simulink model "multi_casadi_robot"  (R2019b)
settings: Solver=FixedStepAuto  StartTime=0.0  StopTime=100  RelTol=1e-3
settings Model: Creator=sanim  LastModifiedBy=Dell
settings DataIOCC: ReturnWorkspaceOutputs=off
settings DebuggingCC: ArithmeticOperatorsInVariantConditions=warning
settings SFSimCC: CustomCodeUndefinedFunction=UseInterfaceOnly

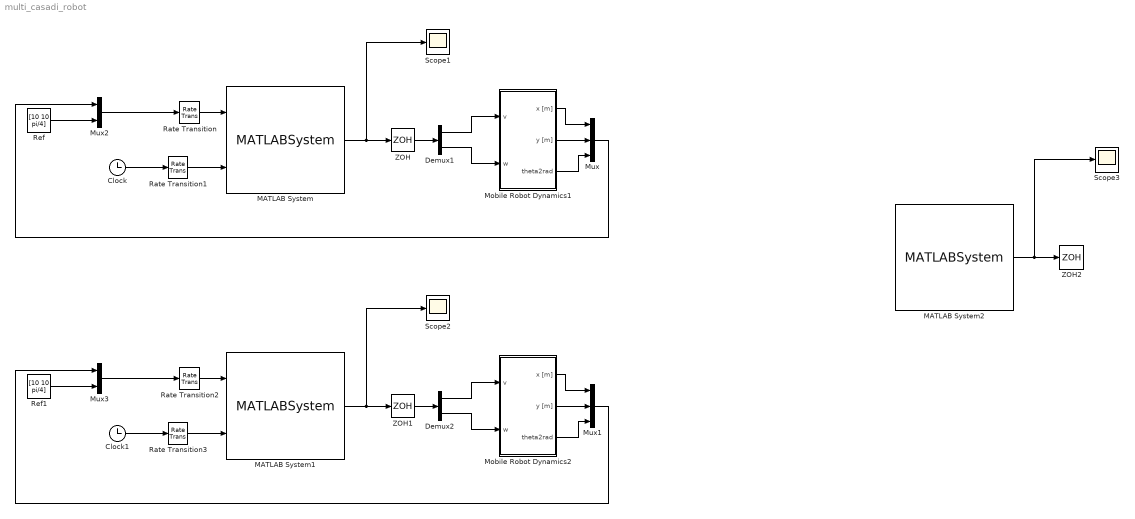
== system multi_casadi_robot ==
  Clock : Clock
  Clock1 : Clock
  Demux1 : Demux  Outputs=2
  Demux2 : Demux  Outputs=2
  MATLAB System : MATLABSystem  System=controller  SimulateUsing=Interpreted execution
      mask Type: controller
      mask Display:
      | disp('controller');
      | port_label('input',1,'x');
      | port_label('input',2,'t');
      | port_label('output',1,'u');
  MATLAB System1 : MATLABSystem  System=controller  SimulateUsing=Interpreted execution
      mask Type: controller
      mask Display:
      | disp('controller');
      | port_label('input',1,'x');
      | port_label('input',2,'t');
      | port_label('output',1,'u');
  MATLAB System2 : MATLABSystem  System=controller  SimulateUsing=Interpreted execution
      mask Type: controller
      mask Display:
      | disp('controller');
      | port_label('input',1,'x');
      | port_label('input',2,'t');
      | port_label('output',1,'u');
  Mobile Robot Dynamics1 : Subsystem
  Mobile Robot Dynamics2 : Subsystem
  Mux : Mux  Inputs=3
  Mux1 : Mux  Inputs=3
  Mux2 : Mux  Inputs=2
  Mux3 : Mux  Inputs=2
  Rate Transition{,1..3} (4 alike) : RateTransition  OutPortSampleTime=0.5
  Ref : Constant  Value=[10 10 pi/4]
  Ref1 : Constant  Value=[10 10 pi/4]
  Scope1 : Scope
  Scope2 : Scope
  Scope3 : Scope
  ZOH : ZeroOrderHold  SampleTime=0.5
  ZOH1 : ZeroOrderHold  SampleTime=0.5
  ZOH2 : ZeroOrderHold  SampleTime=0.5
  wires:
  Mobile Robot Dynamics1/2(y [m]) -> Mux/2
  ZOH/1 -> Demux1/1
  Mux/1 -> Mux2/1
  Ref/1 -> Mux2/2
  Rate Transition/1 -> MATLAB System/1
  MATLAB System/1 -> Scope1/1, ZOH/1
  Demux1/1 -> Mobile Robot Dynamics1/1(v)
  Mobile Robot Dynamics1/3(theta2rad) -> Mux/3
  Mobile Robot Dynamics1/1(x [m]) -> Mux/1
  Rate Transition1/1 -> MATLAB System/2
  Demux1/2 -> Mobile Robot Dynamics1/2(w)
  Clock/1 -> Rate Transition1/1
  Mux2/1 -> Rate Transition/1
  ZOH1/1 -> Demux2/1
  Clock1/1 -> Rate Transition3/1
  Ref1/1 -> Mux3/2
  MATLAB System1/1 -> Scope2/1, ZOH1/1
  Mobile Robot Dynamics2/1(x [m]) -> Mux1/1
  Demux2/1 -> Mobile Robot Dynamics2/1(v)
  Mobile Robot Dynamics2/3(theta2rad) -> Mux1/3
  Mux3/1 -> Rate Transition2/1
  Mux1/1 -> Mux3/1
  Rate Transition2/1 -> MATLAB System1/1
  Rate Transition3/1 -> MATLAB System1/2
  Mobile Robot Dynamics2/2(y [m]) -> Mux1/2
  Demux2/2 -> Mobile Robot Dynamics2/2(w)
  MATLAB System2/1 -> Scope3/1, ZOH2/1

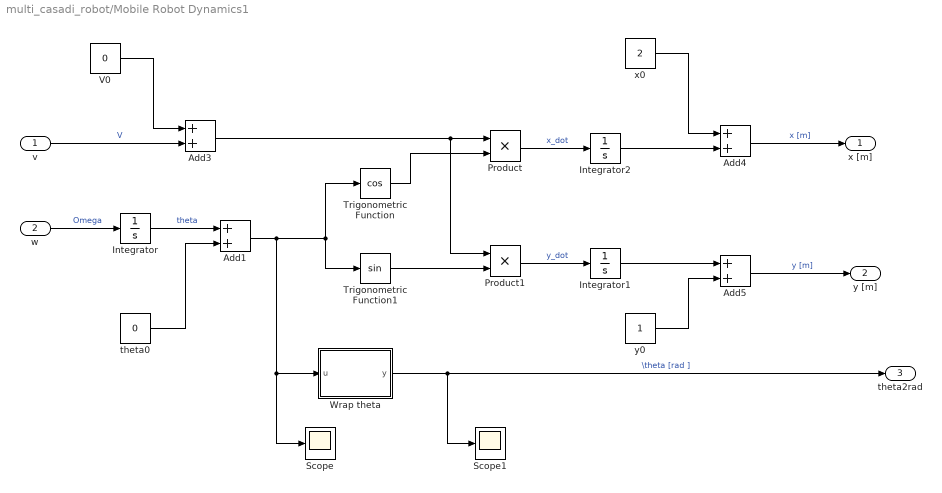
== system multi_casadi_robot/Mobile Robot Dynamics1 ==
  v : Inport
  w : Inport  Port=2
  Add{1,3..5} (4 alike) : Sum
  Integrator : Integrator
  Integrator1 : Integrator
  Integrator2 : Integrator
  Product : Product
  Product1 : Product
  Scope : Scope
  Scope1 : Scope
  Trigonometric Function : Trigonometry  Operator=cos
  Trigonometric Function1 : Trigonometry
  "V0 " : Constant  Value=0
  Wrap theta : MATLAB Function  TreatAsAtomicUnit=on
  theta0 : Constant  Value=0
  x0 : Constant  Value=2
  y0 : Constant
  x [m] : Outport  VectorParamsAs1DForOutWhenUnconnected=off
  y [m] : Outport  Port=2  VectorParamsAs1DForOutWhenUnconnected=off
  theta2rad : Outport  Port=3  VectorParamsAs1DForOutWhenUnconnected=off
  wires:
  w/1 -> Integrator/1  "Omega"
  x0/1 -> Add4/1
  Product1/1 -> Integrator1/1  "y_dot"
  v/1 -> Add3/2  "V"
  theta0/1 -> Add1/2
  Trigonometric Function/1 -> Product/2
  Integrator2/1 -> Add4/2
  Add3/1 -> Product/1, Product1/1
  Add5/1 -> y [m]/1  "y [m]"
  Add4/1 -> x [m]/1  "x [m]"
  Integrator/1 -> Add1/1  "theta"
  Trigonometric Function1/1 -> Product1/2
  y0/1 -> Add5/2
  Product/1 -> Integrator2/1  "x_dot"
  Wrap theta/1(y) -> theta2rad/1, Scope1/1  "\\theta [rad ]"
  "V0 "/1 -> Add3/1
  Integrator1/1 -> Add5/1
  Add1/1 -> Trigonometric Function/1, Trigonometric Function1/1, Scope/1, Wrap theta/1(u)

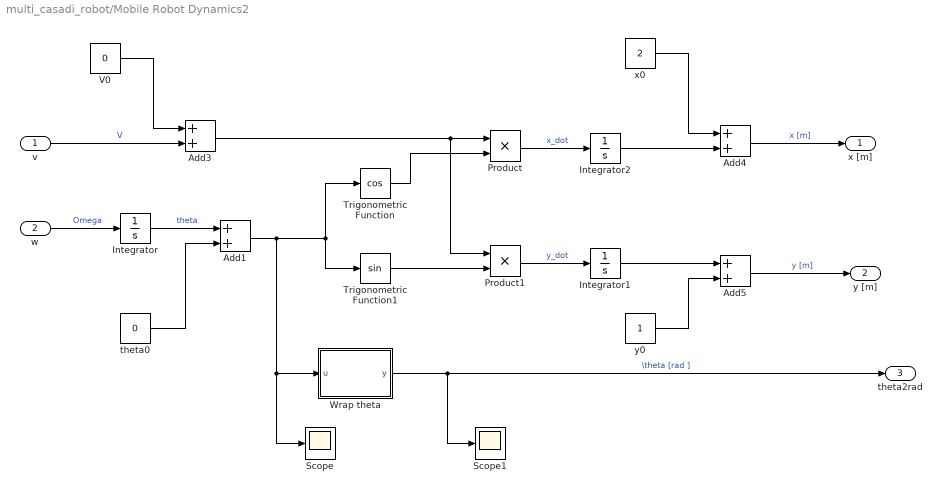
== system multi_casadi_robot/Mobile Robot Dynamics2 ==
  v : Inport
  w : Inport  Port=2
  Add{1,3..5} (4 alike) : Sum
  Integrator : Integrator
  Integrator1 : Integrator
  Integrator2 : Integrator
  Product : Product
  Product1 : Product
  Scope : Scope
  Scope1 : Scope
  Trigonometric Function : Trigonometry  Operator=cos
  Trigonometric Function1 : Trigonometry
  "V0 " : Constant  Value=0
  Wrap theta : MATLAB Function  TreatAsAtomicUnit=on
  theta0 : Constant  Value=0
  x0 : Constant  Value=2
  y0 : Constant
  x [m] : Outport  VectorParamsAs1DForOutWhenUnconnected=off
  y [m] : Outport  Port=2  VectorParamsAs1DForOutWhenUnconnected=off
  theta2rad : Outport  Port=3  VectorParamsAs1DForOutWhenUnconnected=off
  wires:
  w/1 -> Integrator/1  "Omega"
  x0/1 -> Add4/1
  Product1/1 -> Integrator1/1  "y_dot"
  v/1 -> Add3/2  "V"
  theta0/1 -> Add1/2
  Trigonometric Function/1 -> Product/2
  Integrator2/1 -> Add4/2
  Add3/1 -> Product/1, Product1/1
  Add5/1 -> y [m]/1  "y [m]"
  Add4/1 -> x [m]/1  "x [m]"
  Integrator/1 -> Add1/1  "theta"
  Trigonometric Function1/1 -> Product1/2
  y0/1 -> Add5/2
  Product/1 -> Integrator2/1  "x_dot"
  Wrap theta/1(y) -> theta2rad/1, Scope1/1  "\\theta [rad ]"
  "V0 "/1 -> Add3/1
  Integrator1/1 -> Add5/1
  Add1/1 -> Trigonometric Function/1, Trigonometric Function1/1, Scope/1, Wrap theta/1(u)

== matlab function multi_casadi_robot/Mobile Robot Dynamics1/Wrap theta ==
  data: u input; y output
function y = Theta(u)
%#codegen

positiveInput = (u > 0);
y = mod(u, 2*pi);
y((u == 0) & positiveInput) = 2*pi;

== matlab function multi_casadi_robot/Mobile Robot Dynamics2/Wrap theta ==
  data: u input; y output
function y = Theta(u)
%#codegen

positiveInput = (u > 0);
y = mod(u, 2*pi);
y((u == 0) & positiveInput) = 2*pi;
